simulink model "motor_model_23b"  (R2023b)
settings: Solver=VariableStepAuto  StartTime=0.0  StopTime=2  RelTol=1e-3
values from neighbouring files (symbols this model uses):
  D = 8.57e-7    (= 8.57e-07)    [motor_model_m.m]    (also in sampling_exercise.m)
  J = 0.94e-6    (= 9.4e-07)    [motor_model_m.m]    (also in sampling_exercise.m)
  Kb = Kt    (= 0.008863)    [motor_model_m.m]    (also in sampling_exercise.m)
  Kt = 0.008863    [motor_model_m.m]    (also in sampling_exercise.m)
  L = 3.57e-3    (= 0.00357)    [motor_model_m.m]    (also in sampling_exercise.m)
  R = 3.57    [motor_model_m.m]    (also in sampling_exercise.m)
  r2m = wheelRadius/gear    (= 0.00309917355372)    [motor_model_m.m]    (also in sampling_exercise.m = 0.003125)
settings Model: Creator=chr  LastModifiedBy=chr
settings RTWCC: GPUComputeCapability=5.0

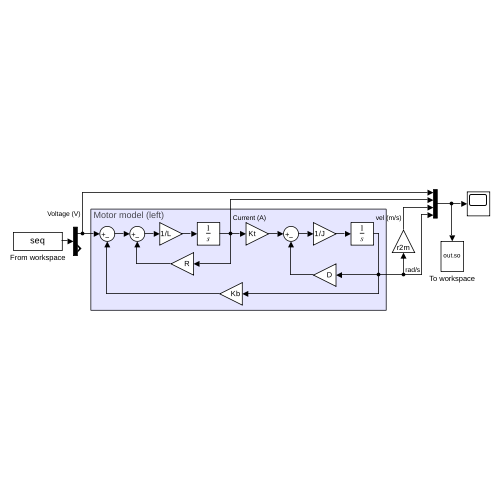
[thumbnail: Simulink's stored preview of the top-level diagram]
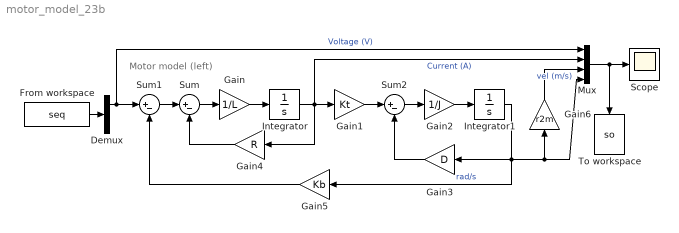
== system motor_model_23b ==
  note: Motor model (left)
  Demux : Demux  Outputs=2
  From workspace : FromWorkspace  VariableName=seq  SampleTime=0.0005  Interpolate=off  OutputAfterFinalValue=Setting to zero
  Gain : Gain  Gain=1/L
  Gain1 : Gain  Gain=Kt
  Gain2 : Gain  Gain=1/J
  Gain3 : Gain  Gain=D
  Gain4 : Gain  Gain=R
  Gain5 : Gain  Gain=Kb
  Gain6 : Gain  Gain=r2m
  Integrator : Integrator
  Integrator1 : Integrator
  Mux : Mux
  Scope : Scope
  Sum : Sum  Inputs=|+-
  Sum1 : Sum  Inputs=|+-
  Sum2 : Sum  Inputs=|+-
  To workspace : ToWorkspace  VariableName=so  SaveFormat=Timeseries  SampleTime=-1
  wires:
  Gain/1 -> Integrator/1
  Sum/1 -> Gain/1
  Integrator/1 -> Mux/2, Gain4/1, Gain1/1  "Current (A)"
  Sum1/1 -> Sum/1
  Gain1/1 -> Sum2/1
  Sum2/1 -> Gain2/1
  Gain2/1 -> Integrator1/1
  Integrator1/1 -> Gain3/1, Gain5/1, Gain6/1, Mux/4  "rad/s"
  Gain3/1 -> Sum2/2
  Gain4/1 -> Sum/2
  Gain5/1 -> Sum1/2
  From workspace/1 -> Demux/1
  Mux/1 -> Scope/1, To workspace/1
  Gain6/1 -> Mux/3  "vel (m/s)"
  Demux/1 -> Mux/1, Sum1/1  "Voltage (V)"
